simulink model "SynRM"  (Simulink 7.7)
settings: Solver=ode45  StartTime=0.0  StopTime=10  RelTol=1e-3
settings Model: Creator=Sayed  LastModifiedBy=Sayed

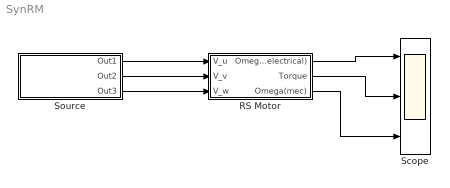
== system SynRM ==
  RS Motor : Subsystem
  Scope : Scope  NumInputPorts=3
      settings: YMin=0~-5~-5  YMax=14~5~5
  "Source " : Subsystem
  wires:
  "Source "/1(Out1) -> RS Motor/1(V_u)
  "Source "/2(Out2) -> RS Motor/2(V_v)
  "Source "/3(Out3) -> RS Motor/3(V_w)
  RS Motor/1(Omega(electrical)) -> Scope/1
  RS Motor/2(Torque) -> Scope/2
  RS Motor/3(Omega(mec)) -> Scope/3

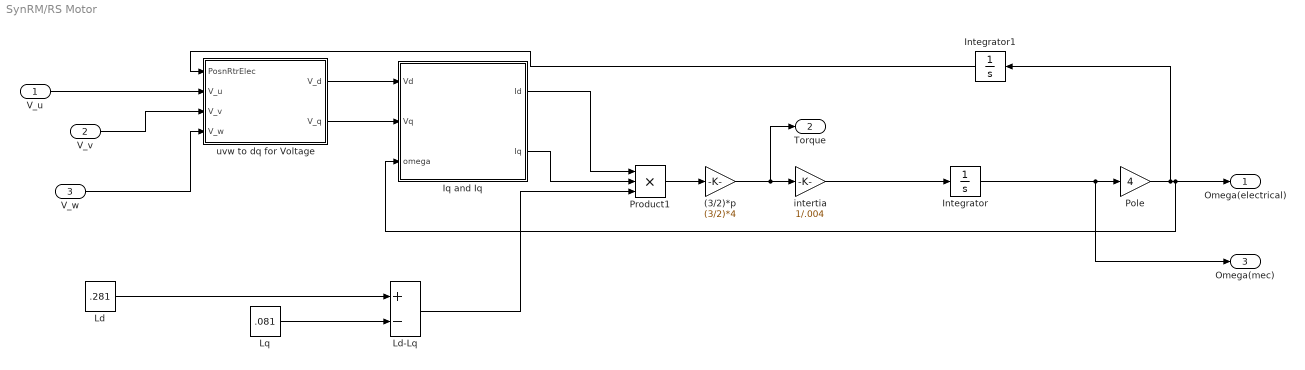
== system SynRM/RS Motor ==
  V_u : Inport
  V_v : Inport  Port=2
  V_w : Inport  Port=3
  (3/2)*p : Gain  Gain=(3/2)*4
  Integrator : Integrator
  Integrator1 : Integrator
  Iq and Iq : Subsystem
  Ld : Constant  Value=.281
  Ld-Lq : Sum  Inputs=+-
  Lq : Constant  Value=.081
  Pole : Gain  Gain=4
  Product1 : Product  Inputs=3  RndMeth=Zero
  intertia : Gain  Gain=1/.004
  uvw to dq for Voltage : Subsystem
  Omega(electrical) : Outport
  Torque : Outport  Port=2
  Omega(mec) : Outport  Port=3
  wires:
  V_u/1 -> uvw to dq for Voltage/2(V_u)
  Ld/1 -> Ld-Lq/1
  Lq/1 -> Ld-Lq/2
  uvw to dq for Voltage/1(V_d) -> Iq and Iq/1(Vd)
  uvw to dq for Voltage/2(V_q) -> Iq and Iq/2(Vq)
  Iq and Iq/1(Id) -> Product1/1
  Iq and Iq/2(Iq) -> Product1/2
  Ld-Lq/1 -> Product1/3
  Product1/1 -> (3/2)*p/1
  (3/2)*p/1 -> Torque/1, intertia/1
  Pole/1 -> Integrator1/1, Omega(electrical)/1, Iq and Iq/3(omega)
  Integrator/1 -> Pole/1, Omega(mec)/1
  intertia/1 -> Integrator/1
  V_v/1 -> uvw to dq for Voltage/3(V_v)
  V_w/1 -> uvw to dq for Voltage/4(V_w)
  Integrator1/1 -> uvw to dq for Voltage/1(PosnRtrElec)

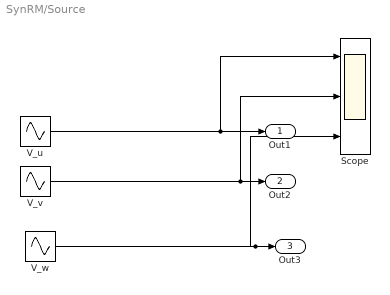
== system SynRM/Source  ==
  Scope : Scope  NumInputPorts=3
      settings: YMin=0~-5~-5  YMax=14~5~5  SaveName=ScopeData3
  V_u : Sin  Amplitude=220  Frequency=100  SampleTime=0
  V_v : Sin  Amplitude=220  Frequency=100  Phase=(2*pi)/3  SampleTime=0
  V_w : Sin  Amplitude=220  Frequency=100  Phase=(4*pi)/3  SampleTime=0
  Out1 : Outport
  Out2 : Outport  Port=2
  Out3 : Outport  Port=3
  wires:
  V_u/1 -> Out1/1, Scope/1
  V_v/1 -> Out2/1, Scope/2
  V_w/1 -> Out3/1, Scope/3

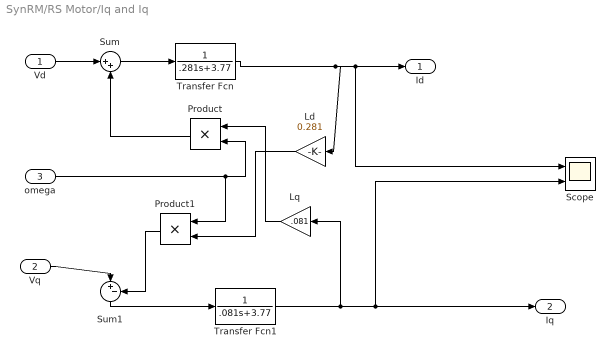
== system SynRM/RS Motor/Iq and Iq ==
  Vd : Inport
  Vq : Inport  Port=2
  omega : Inport  Port=3
  Ld : Gain  Gain=0.281
  Lq : Gain  Gain=.081
  Product : Product  RndMeth=Zero
  Product1 : Product  RndMeth=Zero
  Scope : Scope  NumInputPorts=2
      settings: TimeRange=0.0711550339715874  YMin=-5~-0.4952941176470587  YMax=5~1.410588235294118  SaveName=ScopeData2
  Sum : Sum  Inputs=|++
  Sum1 : Sum  Inputs=|+-
  Transfer Fcn : TransferFcn  Denominator=[.281 3.77]
  Transfer Fcn1 : TransferFcn  Denominator=[.081 3.77]
  Id : Outport
  Iq : Outport  Port=2
  wires:
  Transfer Fcn/1 -> Id/1, Scope/1, Ld/1
  Vd/1 -> Sum/1
  Sum/1 -> Transfer Fcn/1
  Lq/1 -> Product/1
  omega/1 -> Product/2, Product1/1
  Product/1 -> Sum/2
  Ld/1 -> Product1/2
  Vq/1 -> Sum1/1
  Product1/1 -> Sum1/2
  Sum1/1 -> Transfer Fcn1/1
  Transfer Fcn1/1 -> Iq/1, Scope/2, Lq/1

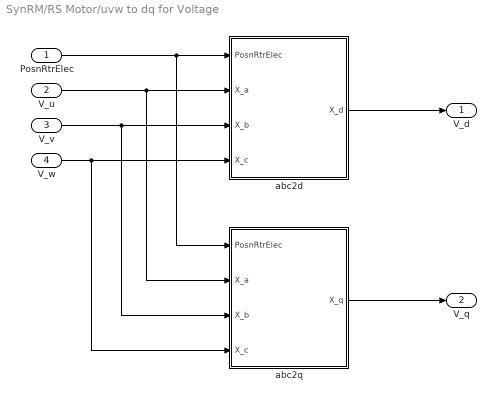
== system SynRM/RS Motor/uvw to dq for Voltage ==
  PosnRtrElec : Inport
  V_u : Inport  Port=2
  V_v : Inport  Port=3
  V_w : Inport  Port=4
  abc2d : Subsystem
  abc2q : Subsystem
  V_d : Outport
  V_q : Outport  Port=2
  wires:
  PosnRtrElec/1 -> abc2d/1(PosnRtrElec), abc2q/1(PosnRtrElec)
  V_u/1 -> abc2d/2(X_a), abc2q/2(X_a)
  V_v/1 -> abc2d/3(X_b), abc2q/3(X_b)
  V_w/1 -> abc2d/4(X_c), abc2q/4(X_c)
  abc2d/1(X_d) -> V_d/1
  abc2q/1(X_q) -> V_q/1

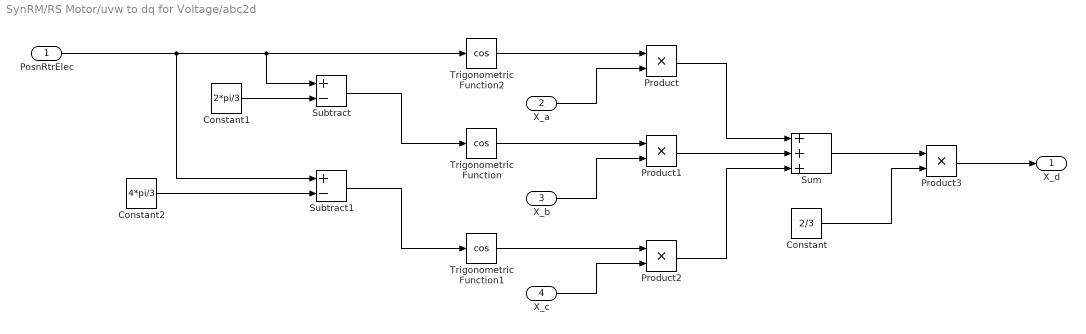
== system SynRM/RS Motor/uvw to dq for Voltage/abc2d ==
  PosnRtrElec : Inport
  X_a : Inport  Port=2
  X_b : Inport  Port=3
  X_c : Inport  Port=4
  Constant : Constant  Value=2/3
  Constant1 : Constant  Value=2*pi/3
  Constant2 : Constant  Value=4*pi/3
  Product{,1..3} (4 alike) : Product  RndMeth=Zero
  Subtract : Sum  Inputs=+-
  Subtract1 : Sum  Inputs=+-
  Sum : Sum  Inputs=+++
  Trigonometric Function : Trigonometry  Operator=cos
  Trigonometric Function1 : Trigonometry  Operator=cos
  Trigonometric Function2 : Trigonometry  Operator=cos
  X_d : Outport
  wires:
  PosnRtrElec/1 -> Subtract1/1, Trigonometric Function2/1, Subtract/1
  Constant1/1 -> Subtract/2
  Constant2/1 -> Subtract1/2
  Subtract/1 -> Trigonometric Function/1
  Subtract1/1 -> Trigonometric Function1/1
  Trigonometric Function2/1 -> Product/1
  Trigonometric Function/1 -> Product1/1
  Trigonometric Function1/1 -> Product2/1
  X_a/1 -> Product/2
  X_b/1 -> Product1/2
  X_c/1 -> Product2/2
  Product/1 -> Sum/1
  Product1/1 -> Sum/2
  Product2/1 -> Sum/3
  Sum/1 -> Product3/1
  Constant/1 -> Product3/2
  Product3/1 -> X_d/1

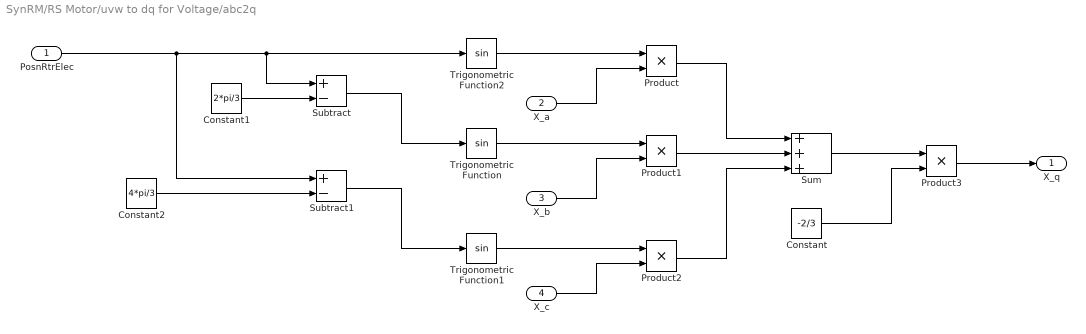
== system SynRM/RS Motor/uvw to dq for Voltage/abc2q ==
  PosnRtrElec : Inport
  X_a : Inport  Port=2
  X_b : Inport  Port=3
  X_c : Inport  Port=4
  Constant : Constant  Value=-2/3
  Constant1 : Constant  Value=2*pi/3
  Constant2 : Constant  Value=4*pi/3
  Product{,1..3} (4 alike) : Product  RndMeth=Zero
  Subtract : Sum  Inputs=+-
  Subtract1 : Sum  Inputs=+-
  Sum : Sum  Inputs=+++
  Trigonometric Function : Trigonometry
  Trigonometric Function1 : Trigonometry
  Trigonometric Function2 : Trigonometry
  X_q : Outport
  wires:
  Product3/1 -> X_q/1
  Constant/1 -> Product3/2
  Sum/1 -> Product3/1
  Product2/1 -> Sum/3
  Product1/1 -> Sum/2
  Product/1 -> Sum/1
  X_c/1 -> Product2/2
  X_b/1 -> Product1/2
  X_a/1 -> Product/2
  Trigonometric Function1/1 -> Product2/1
  Trigonometric Function/1 -> Product1/1
  Trigonometric Function2/1 -> Product/1
  Subtract1/1 -> Trigonometric Function1/1
  Subtract/1 -> Trigonometric Function/1
  Constant2/1 -> Subtract1/2
  Constant1/1 -> Subtract/2
  PosnRtrElec/1 -> Subtract/1, Trigonometric Function2/1, Subtract1/1
